simulink model "c00006M_harness"  (R2018a)
settings: Solver=FixedStepAuto  StartTime=0.0  StopTime=300  FixedStep=0.1  RelTol=1e-3
undefined symbols (not defined in the file): A1, hmax, PriorityTank, R1, R2, sigbuilder_block, TempThreshold
(part 19 of 66)

== system c00006M_harness/M091/Tank3/Control ==
  note: 1: Maintenance
      | 2: Reference
      | 3: Manual
  ControlType : Inport
  StartMaintenance : Inport  Port=2
  ManualReference : Inport  Port=3
  Fill : Inport  Port=4
  Empty : Inport  Port=5
  EmergencyButton : Inport  Port=6
  Temperature : Inport  Port=7
  LiquidLevel : Inport  Port=8
  Constant : Constant  Value=0
  Constant1 : Constant  Value=TempThreshold
  Logical Operator : Logic  Operator=OR  AllPortsSameDT=off  OutDataTypeStr=boolean
  Logical Operator1 : Logic  Operator=OR  AllPortsSameDT=off  OutDataTypeStr=boolean
  Maintenance : Subsystem
  ManualControlLiquidInOut : Subsystem
  ManualControlReference : Subsystem
  Multiport Switch : MultiPortSwitch
  Multiport Switch1 : MultiPortSwitch
  Relational Operator : RelationalOperator  Operator=>  OutDataTypeStr=boolean  RndMeth=Simplest
  Switch : Switch  Criteria=u2 > Threshold
  Switch1 : Switch  Criteria=u2 > Threshold
  LiquidIn : Outport
  LiquidOut : Outport  Port=2
  wires:
  Multiport Switch/1 -> Switch/3
  Multiport Switch1/1 -> Switch1/3
  ControlType/1 -> Multiport Switch1/1, Multiport Switch/1, Maintenance/1(Type)
  Maintenance/1(LiquidIn) -> Multiport Switch/2
  ManualControlReference/1(LiquidIn) -> Multiport Switch/3
  Maintenance/2(LiquidOut) -> Multiport Switch1/2
  ManualControlReference/2(LiquidOut) -> Multiport Switch1/3
  ManualReference/1 -> ManualControlReference/1(ManualReference)
  LiquidLevel/1 -> ManualControlLiquidInOut/3(LiquidLevel), ManualControlReference/2(LiquidLevel), Maintenance/3(LiquidLevel)
  ManualControlLiquidInOut/1(LiquidIn) -> Multiport Switch/4
  ManualControlLiquidInOut/2(LiquidOut) -> Multiport Switch1/4
  Empty/1 -> ManualControlLiquidInOut/2(Empty)
  Fill/1 -> ManualControlLiquidInOut/1(Fill)
  StartMaintenance/1 -> Maintenance/2(StartMaintenance)
  Switch/1 -> LiquidIn/1
  Switch1/1 -> LiquidOut/1
  Constant/1 -> Switch1/1, Switch/1
  EmergencyButton/1 -> Logical Operator/1, Logical Operator1/1
  Relational Operator/1 -> Logical Operator1/2, Logical Operator/2
  Logical Operator/1 -> Switch1/2
  Logical Operator1/1 -> Switch/2
  Temperature/1 -> Relational Operator/1
  Constant1/1 -> Relational Operator/2

== system c00006M_harness/M091/Tank3/MasterTankControl ==
  note: Priority tank must always have more liquid than others
  LiquidTank2 : Inport
  LiquidTank3 : Inport  Port=2
  Constant : Constant  Value=PriorityTank
  Constant1 : Constant  Value=false
  Logical Operator : Logic  Operator=NOT  AllPortsSameDT=off  OutDataTypeStr=boolean
  Multiport Switch : MultiPortSwitch
  Relational Operator1 : RelationalOperator  OutDataTypeStr=boolean  RndMeth=Simplest
  AllowTheTankFilling : Outport
  wires:
  Constant/1 -> Multiport Switch/1
  Relational Operator1/1 -> Multiport Switch/3
  Constant1/1 -> Multiport Switch/4, Multiport Switch/2
  Multiport Switch/1 -> Logical Operator/1
  Logical Operator/1 -> AllowTheTankFilling/1
  LiquidTank2/1 -> Relational Operator1/2
  LiquidTank3/1 -> Relational Operator1/1

== system c00006M_harness/M091/Tank3/TankModel ==
  LiquidIn : Inport
  LiquidOut : Inport  Port=2
  Add1 : Sum  Inputs=+-
  Constant1 : Constant  Value=0
  Constant2 : Constant  Value=0
  Constant3 : Constant
  Gain : Gain  Gain=1/R1
  Gain1 : Gain  Gain=1/A1
  Gain2 : Gain  Gain=1/R2
  Integrator : Integrator
  Saturation : Saturate  UpperLimit=hmax  LowerLimit=0
  Switch : Switch  Criteria=u2 ~= 0
  Switch1 : Switch  Criteria=u2 ~= 0
  LiquidLevel : Outport
  wires:
  Saturation/1 -> LiquidLevel/1, Gain2/1
  LiquidOut/1 -> Switch/2
  Add1/1 -> Gain1/1
  Gain2/1 -> Switch/1
  LiquidIn/1 -> Switch1/2
  Switch/1 -> Add1/2
  Switch1/1 -> Gain/1
  Constant2/1 -> Switch/3
  Constant3/1 -> Switch1/1
  Integrator/1 -> Saturation/1
  Gain1/1 -> Integrator/1
  Gain/1 -> Add1/1
  Constant1/1 -> Switch1/3

== system c00006M_harness/M092/Tank2/Control ==
  note: 1: Maintenance
      | 2: Reference
      | 3: Manual
  ControlType : Inport
  StartMaintenance : Inport  Port=2
  ManualReference : Inport  Port=3
  Fill : Inport  Port=4
  Empty : Inport  Port=5
  EmergencyButton : Inport  Port=6
  Temperature : Inport  Port=7
  LiquidLevel : Inport  Port=8
  Constant : Constant  Value=0
  Constant1 : Constant  Value=TempThreshold
  Logical Operator : Logic  Operator=OR  AllPortsSameDT=off  OutDataTypeStr=boolean
  Logical Operator1 : Logic  Operator=OR  AllPortsSameDT=off  OutDataTypeStr=boolean
  Maintenance : Subsystem
  ManualControlLiquidInOut : Subsystem
  ManualControlReference : Subsystem
  Multiport Switch : MultiPortSwitch
  Multiport Switch1 : MultiPortSwitch
  Relational Operator : RelationalOperator  Operator=>  OutDataTypeStr=boolean  RndMeth=Simplest
  Switch : Switch  Criteria=u2 > Threshold
  Switch1 : Switch  Criteria=u2 > Threshold
  LiquidIn : Outport
  LiquidOut : Outport  Port=2
  wires:
  Multiport Switch/1 -> Switch/3
  Multiport Switch1/1 -> Switch1/3
  ControlType/1 -> Multiport Switch1/1, Multiport Switch/1, Maintenance/1(Type)
  Maintenance/1(LiquidIn) -> Multiport Switch/2
  ManualControlReference/1(LiquidIn) -> Multiport Switch/3
  Maintenance/2(LiquidOut) -> Multiport Switch1/2
  ManualControlReference/2(LiquidOut) -> Multiport Switch1/3
  ManualReference/1 -> ManualControlReference/1(ManualReference)
  LiquidLevel/1 -> ManualControlLiquidInOut/3(LiquidLevel), ManualControlReference/2(LiquidLevel), Maintenance/3(LiquidLevel)
  ManualControlLiquidInOut/1(LiquidIn) -> Multiport Switch/4
  ManualControlLiquidInOut/2(LiquidOut) -> Multiport Switch1/4
  Empty/1 -> ManualControlLiquidInOut/2(Empty)
  Fill/1 -> ManualControlLiquidInOut/1(Fill)
  StartMaintenance/1 -> Maintenance/2(StartMaintenance)
  Switch/1 -> LiquidIn/1
  Switch1/1 -> LiquidOut/1
  Constant/1 -> Switch1/1, Switch/1
  EmergencyButton/1 -> Logical Operator/1, Logical Operator1/1
  Relational Operator/1 -> Logical Operator1/2, Logical Operator/2
  Logical Operator/1 -> Switch1/2
  Logical Operator1/1 -> Switch/2
  Temperature/1 -> Relational Operator/1
  Constant1/1 -> Relational Operator/2

== system c00006M_harness/M092/Tank2/MasterTankControl ==
  note: Priority tank must always have more liquid than others
  LiquidTank2 : Inport
  LiquidTank3 : Inport  Port=2
  Constant : Constant  Value=PriorityTank
  Constant1 : Constant  Value=false
  Logical Operator : Logic  Operator=NOT  AllPortsSameDT=off  OutDataTypeStr=boolean
  Multiport Switch : MultiPortSwitch
  Relational Operator1 : RelationalOperator  OutDataTypeStr=boolean  RndMeth=Simplest
  AllowTheTankFilling : Outport
  wires:
  LiquidTank2/1 -> Relational Operator1/1
  LiquidTank3/1 -> Relational Operator1/2
  Constant/1 -> Multiport Switch/1
  Relational Operator1/1 -> Multiport Switch/4
  Constant1/1 -> Multiport Switch/3, Multiport Switch/2
  Multiport Switch/1 -> Logical Operator/1
  Logical Operator/1 -> AllowTheTankFilling/1

== system c00006M_harness/M092/Tank2/TankModel ==
  LiquidIn : Inport
  LiquidOut : Inport  Port=2
  Add1 : Sum  Inputs=+-
  Constant1 : Constant  Value=0
  Constant2 : Constant  Value=0
  Constant3 : Constant
  Gain : Gain  Gain=1/R1
  Gain1 : Gain  Gain=1/A1
  Gain2 : Gain  Gain=1/R2
  Integrator : Integrator
  Saturation : Saturate  UpperLimit=hmax  LowerLimit=0
  Switch : Switch  Criteria=u2 ~= 0
  Switch1 : Switch  Criteria=u2 ~= 0
  LiquidLevel : Outport
  wires:
  Saturation/1 -> LiquidLevel/1, Gain2/1
  LiquidOut/1 -> Switch/2
  Add1/1 -> Gain1/1
  Gain2/1 -> Switch/1
  LiquidIn/1 -> Switch1/2
  Switch/1 -> Add1/2
  Switch1/1 -> Gain/1
  Constant2/1 -> Switch/3
  Constant3/1 -> Switch1/1
  Integrator/1 -> Saturation/1
  Gain1/1 -> Integrator/1
  Gain/1 -> Add1/1
  Constant1/1 -> Switch1/3

== system c00006M_harness/M092/Tank3/Control ==
  note: 1: Maintenance
      | 2: Reference
      | 3: Manual
  ControlType : Inport
  StartMaintenance : Inport  Port=2
  ManualReference : Inport  Port=3
  Fill : Inport  Port=4
  Empty : Inport  Port=5
  EmergencyButton : Inport  Port=6
  Temperature : Inport  Port=7
  LiquidLevel : Inport  Port=8
  Constant : Constant  Value=0
  Constant1 : Constant  Value=TempThreshold
  Logical Operator : Logic  Operator=OR  AllPortsSameDT=off  OutDataTypeStr=boolean
  Logical Operator1 : Logic  Operator=OR  AllPortsSameDT=off  OutDataTypeStr=boolean
  Maintenance : Subsystem
  ManualControlLiquidInOut : Subsystem
  ManualControlReference : Subsystem
  Multiport Switch : MultiPortSwitch
  Multiport Switch1 : MultiPortSwitch
  Relational Operator : RelationalOperator  Operator=>  OutDataTypeStr=boolean  RndMeth=Simplest
  Switch : Switch  Criteria=u2 > Threshold
  Switch1 : Switch  Criteria=u2 > Threshold
  LiquidIn : Outport
  LiquidOut : Outport  Port=2
  wires:
  Multiport Switch/1 -> Switch/3
  Multiport Switch1/1 -> Switch1/3
  ControlType/1 -> Multiport Switch1/1, Multiport Switch/1, Maintenance/1(Type)
  Maintenance/1(LiquidIn) -> Multiport Switch/2
  ManualControlReference/1(LiquidIn) -> Multiport Switch/3
  Maintenance/2(LiquidOut) -> Multiport Switch1/2
  ManualControlReference/2(LiquidOut) -> Multiport Switch1/3
  ManualReference/1 -> ManualControlReference/1(ManualReference)
  LiquidLevel/1 -> ManualControlLiquidInOut/3(LiquidLevel), ManualControlReference/2(LiquidLevel), Maintenance/3(LiquidLevel)
  ManualControlLiquidInOut/1(LiquidIn) -> Multiport Switch/4
  ManualControlLiquidInOut/2(LiquidOut) -> Multiport Switch1/4
  Empty/1 -> ManualControlLiquidInOut/2(Empty)
  Fill/1 -> ManualControlLiquidInOut/1(Fill)
  StartMaintenance/1 -> Maintenance/2(StartMaintenance)
  Switch/1 -> LiquidIn/1
  Switch1/1 -> LiquidOut/1
  Constant/1 -> Switch1/1, Switch/1
  EmergencyButton/1 -> Logical Operator/1, Logical Operator1/1
  Relational Operator/1 -> Logical Operator1/2, Logical Operator/2
  Logical Operator/1 -> Switch1/2
  Logical Operator1/1 -> Switch/2
  Temperature/1 -> Relational Operator/1
  Constant1/1 -> Relational Operator/2

== system c00006M_harness/M092/Tank3/MasterTankControl ==
  note: Priority tank must always have more liquid than others
  LiquidTank2 : Inport
  LiquidTank3 : Inport  Port=2
  Constant : Constant  Value=PriorityTank
  Constant1 : Constant  Value=false
  Logical Operator : Logic  Operator=NOT  AllPortsSameDT=off  OutDataTypeStr=boolean
  Multiport Switch : MultiPortSwitch
  Relational Operator1 : RelationalOperator  OutDataTypeStr=boolean  RndMeth=Simplest
  AllowTheTankFilling : Outport
  wires:
  Constant/1 -> Multiport Switch/1
  Relational Operator1/1 -> Multiport Switch/3
  Constant1/1 -> Multiport Switch/4, Multiport Switch/2
  Multiport Switch/1 -> Logical Operator/1
  Logical Operator/1 -> AllowTheTankFilling/1
  LiquidTank2/1 -> Relational Operator1/2
  LiquidTank3/1 -> Relational Operator1/1

== system c00006M_harness/M092/Tank3/TankModel ==
  LiquidIn : Inport
  LiquidOut : Inport  Port=2
  Add1 : Sum  Inputs=+-
  Constant1 : Constant  Value=0
  Constant2 : Constant  Value=0
  Constant3 : Constant
  Gain : Gain  Gain=1/R1
  Gain1 : Gain  Gain=1/A1
  Gain2 : Gain  Gain=1/R2
  Integrator : Integrator
  Saturation : Saturate  UpperLimit=hmax  LowerLimit=0
  Switch : Switch  Criteria=u2 ~= 0
  Switch1 : Switch  Criteria=u2 ~= 0
  LiquidLevel : Outport
  wires:
  Saturation/1 -> LiquidLevel/1, Gain2/1
  LiquidOut/1 -> Switch/2
  Add1/1 -> Gain1/1
  Gain2/1 -> Switch/1
  LiquidIn/1 -> Switch1/2
  Switch/1 -> Add1/2
  Switch1/1 -> Gain/1
  Constant2/1 -> Switch/3
  Constant3/1 -> Switch1/1
  Integrator/1 -> Saturation/1
  Gain1/1 -> Integrator/1
  Gain/1 -> Add1/1
  Constant1/1 -> Switch1/3

== system c00006M_harness/M093/Tank2/Control ==
  note: 1: Maintenance
      | 2: Reference
      | 3: Manual
  ControlType : Inport
  StartMaintenance : Inport  Port=2
  ManualReference : Inport  Port=3
  Fill : Inport  Port=4
  Empty : Inport  Port=5
  EmergencyButton : Inport  Port=6
  Temperature : Inport  Port=7
  LiquidLevel : Inport  Port=8
  Constant : Constant  Value=0
  Constant1 : Constant  Value=TempThreshold
  Logical Operator : Logic  Operator=OR  AllPortsSameDT=off  OutDataTypeStr=boolean
  Logical Operator1 : Logic  Operator=OR  AllPortsSameDT=off  OutDataTypeStr=boolean
  Maintenance : Subsystem
  ManualControlLiquidInOut : Subsystem
  ManualControlReference : Subsystem
  Multiport Switch : MultiPortSwitch
  Multiport Switch1 : MultiPortSwitch
  Relational Operator : RelationalOperator  Operator=>  OutDataTypeStr=boolean  RndMeth=Simplest
  Switch : Switch  Criteria=u2 > Threshold
  Switch1 : Switch  Criteria=u2 > Threshold
  LiquidIn : Outport
  LiquidOut : Outport  Port=2
  wires:
  Multiport Switch/1 -> Switch/3
  Multiport Switch1/1 -> Switch1/3
  ControlType/1 -> Multiport Switch1/1, Multiport Switch/1, Maintenance/1(Type)
  Maintenance/1(LiquidIn) -> Multiport Switch/2
  ManualControlReference/1(LiquidIn) -> Multiport Switch/3
  Maintenance/2(LiquidOut) -> Multiport Switch1/2
  ManualControlReference/2(LiquidOut) -> Multiport Switch1/3
  ManualReference/1 -> ManualControlReference/1(ManualReference)
  LiquidLevel/1 -> ManualControlLiquidInOut/3(LiquidLevel), ManualControlReference/2(LiquidLevel), Maintenance/3(LiquidLevel)
  ManualControlLiquidInOut/1(LiquidIn) -> Multiport Switch/4
  ManualControlLiquidInOut/2(LiquidOut) -> Multiport Switch1/4
  Empty/1 -> ManualControlLiquidInOut/2(Empty)
  Fill/1 -> ManualControlLiquidInOut/1(Fill)
  StartMaintenance/1 -> Maintenance/2(StartMaintenance)
  Switch/1 -> LiquidIn/1
  Switch1/1 -> LiquidOut/1
  Constant/1 -> Switch1/1, Switch/1
  EmergencyButton/1 -> Logical Operator/1, Logical Operator1/1
  Relational Operator/1 -> Logical Operator1/2, Logical Operator/2
  Logical Operator/1 -> Switch1/2
  Logical Operator1/1 -> Switch/2
  Temperature/1 -> Relational Operator/1
  Constant1/1 -> Relational Operator/2

== system c00006M_harness/M093/Tank2/MasterTankControl ==
  note: Priority tank must always have more liquid than others
  LiquidTank2 : Inport
  LiquidTank3 : Inport  Port=2
  Constant : Constant  Value=PriorityTank
  Constant1 : Constant  Value=false
  Logical Operator : Logic  Operator=NOT  AllPortsSameDT=off  OutDataTypeStr=boolean
  Multiport Switch : MultiPortSwitch
  Relational Operator1 : RelationalOperator  OutDataTypeStr=boolean  RndMeth=Simplest
  AllowTheTankFilling : Outport
  wires:
  LiquidTank2/1 -> Relational Operator1/1
  LiquidTank3/1 -> Relational Operator1/2
  Constant/1 -> Multiport Switch/1
  Relational Operator1/1 -> Multiport Switch/4
  Constant1/1 -> Multiport Switch/3, Multiport Switch/2
  Multiport Switch/1 -> Logical Operator/1
  Logical Operator/1 -> AllowTheTankFilling/1

== system c00006M_harness/M093/Tank2/TankModel ==
  LiquidIn : Inport
  LiquidOut : Inport  Port=2
  Add1 : Sum  Inputs=+-
  Constant1 : Constant  Value=0
  Constant2 : Constant  Value=0
  Constant3 : Constant
  Gain : Gain  Gain=1/R1
  Gain1 : Gain  Gain=1/A1
  Gain2 : Gain  Gain=1/R2
  Integrator : Integrator
  Saturation : Saturate  UpperLimit=hmax  LowerLimit=0
  Switch : Switch  Criteria=u2 ~= 0
  Switch1 : Switch  Criteria=u2 ~= 0
  LiquidLevel : Outport
  wires:
  Saturation/1 -> LiquidLevel/1, Gain2/1
  LiquidOut/1 -> Switch/2
  Add1/1 -> Gain1/1
  Gain2/1 -> Switch/1
  LiquidIn/1 -> Switch1/2
  Switch/1 -> Add1/2
  Switch1/1 -> Gain/1
  Constant2/1 -> Switch/3
  Constant3/1 -> Switch1/1
  Integrator/1 -> Saturation/1
  Gain1/1 -> Integrator/1
  Gain/1 -> Add1/1
  Constant1/1 -> Switch1/3

== system c00006M_harness/M093/Tank3/Control ==
  note: 1: Maintenance
      | 2: Reference
      | 3: Manual
  ControlType : Inport
  StartMaintenance : Inport  Port=2
  ManualReference : Inport  Port=3
  Fill : Inport  Port=4
  Empty : Inport  Port=5
  EmergencyButton : Inport  Port=6
  Temperature : Inport  Port=7
  LiquidLevel : Inport  Port=8
  Constant : Constant  Value=0
  Constant1 : Constant  Value=TempThreshold
  Logical Operator : Logic  Operator=OR  AllPortsSameDT=off  OutDataTypeStr=boolean
  Logical Operator1 : Logic  Operator=OR  AllPortsSameDT=off  OutDataTypeStr=boolean
  Maintenance : Subsystem
  ManualControlLiquidInOut : Subsystem
  ManualControlReference : Subsystem
  Multiport Switch : MultiPortSwitch
  Multiport Switch1 : MultiPortSwitch
  Relational Operator : RelationalOperator  Operator=>  OutDataTypeStr=boolean  RndMeth=Simplest
  Switch : Switch  Criteria=u2 > Threshold
  Switch1 : Switch  Criteria=u2 > Threshold
  LiquidIn : Outport
  LiquidOut : Outport  Port=2
  wires:
  Multiport Switch/1 -> Switch/3
  Multiport Switch1/1 -> Switch1/3
  ControlType/1 -> Multiport Switch1/1, Multiport Switch/1, Maintenance/1(Type)
  Maintenance/1(LiquidIn) -> Multiport Switch/2
  ManualControlReference/1(LiquidIn) -> Multiport Switch/3
  Maintenance/2(LiquidOut) -> Multiport Switch1/2
  ManualControlReference/2(LiquidOut) -> Multiport Switch1/3
  ManualReference/1 -> ManualControlReference/1(ManualReference)
  LiquidLevel/1 -> ManualControlLiquidInOut/3(LiquidLevel), ManualControlReference/2(LiquidLevel), Maintenance/3(LiquidLevel)
  ManualControlLiquidInOut/1(LiquidIn) -> Multiport Switch/4
  ManualControlLiquidInOut/2(LiquidOut) -> Multiport Switch1/4
  Empty/1 -> ManualControlLiquidInOut/2(Empty)
  Fill/1 -> ManualControlLiquidInOut/1(Fill)
  StartMaintenance/1 -> Maintenance/2(StartMaintenance)
  Switch/1 -> LiquidIn/1
  Switch1/1 -> LiquidOut/1
  Constant/1 -> Switch1/1, Switch/1
  EmergencyButton/1 -> Logical Operator/1, Logical Operator1/1
  Relational Operator/1 -> Logical Operator1/2, Logical Operator/2
  Logical Operator/1 -> Switch1/2
  Logical Operator1/1 -> Switch/2
  Temperature/1 -> Relational Operator/1
  Constant1/1 -> Relational Operator/2

== system c00006M_harness/M093/Tank3/MasterTankControl ==
  note: Priority tank must always have more liquid than others
  LiquidTank2 : Inport
  LiquidTank3 : Inport  Port=2
  Constant : Constant  Value=PriorityTank
  Constant1 : Constant  Value=false
  Logical Operator : Logic  Operator=NOT  AllPortsSameDT=off  OutDataTypeStr=boolean
  Multiport Switch : MultiPortSwitch
  Relational Operator1 : RelationalOperator  OutDataTypeStr=boolean  RndMeth=Simplest
  AllowTheTankFilling : Outport
  wires:
  Constant/1 -> Multiport Switch/1
  Relational Operator1/1 -> Multiport Switch/3
  Constant1/1 -> Multiport Switch/4, Multiport Switch/2
  Multiport Switch/1 -> Logical Operator/1
  Logical Operator/1 -> AllowTheTankFilling/1
  LiquidTank2/1 -> Relational Operator1/2
  LiquidTank3/1 -> Relational Operator1/1

== system c00006M_harness/M093/Tank3/TankModel ==
  LiquidIn : Inport
  LiquidOut : Inport  Port=2
  Add1 : Sum  Inputs=+-
  Constant1 : Constant  Value=0
  Constant2 : Constant  Value=0
  Constant3 : Constant
  Gain : Gain  Gain=1/R1
  Gain1 : Gain  Gain=1/A1
  Gain2 : Gain  Gain=1/R2
  Integrator : Integrator
  Saturation : Saturate  UpperLimit=hmax  LowerLimit=0
  Switch : Switch  Criteria=u2 ~= 0
  Switch1 : Switch  Criteria=u2 ~= 0
  LiquidLevel : Outport
  wires:
  Saturation/1 -> LiquidLevel/1, Gain2/1
  LiquidOut/1 -> Switch/2
  Add1/1 -> Gain1/1
  Gain2/1 -> Switch/1
  LiquidIn/1 -> Switch1/2
  Switch/1 -> Add1/2
  Switch1/1 -> Gain/1
  Constant2/1 -> Switch/3
  Constant3/1 -> Switch1/1
  Integrator/1 -> Saturation/1
  Gain1/1 -> Integrator/1
  Gain/1 -> Add1/1
  Constant1/1 -> Switch1/3

== system c00006M_harness/M094/Tank2/Control ==
  note: 1: Maintenance
      | 2: Reference
      | 3: Manual
  ControlType : Inport
  StartMaintenance : Inport  Port=2
  ManualReference : Inport  Port=3
  Fill : Inport  Port=4
  Empty : Inport  Port=5
  EmergencyButton : Inport  Port=6
  Temperature : Inport  Port=7
  LiquidLevel : Inport  Port=8
  Constant : Constant  Value=0
  Constant1 : Constant  Value=TempThreshold
  Logical Operator : Logic  Operator=OR  AllPortsSameDT=off  OutDataTypeStr=boolean
  Logical Operator1 : Logic  Operator=OR  AllPortsSameDT=off  OutDataTypeStr=boolean
  Maintenance : Subsystem
  ManualControlLiquidInOut : Subsystem
  ManualControlReference : Subsystem
  Multiport Switch : MultiPortSwitch
  Multiport Switch1 : MultiPortSwitch
  Relational Operator : RelationalOperator  Operator=>  OutDataTypeStr=boolean  RndMeth=Simplest
  Switch : Switch  Criteria=u2 > Threshold
  Switch1 : Switch  Criteria=u2 > Threshold
  LiquidIn : Outport
  LiquidOut : Outport  Port=2
  wires:
  Multiport Switch/1 -> Switch/3
  Multiport Switch1/1 -> Switch1/3
  ControlType/1 -> Multiport Switch1/1, Multiport Switch/1, Maintenance/1(Type)
  Maintenance/1(LiquidIn) -> Multiport Switch/2
  ManualControlReference/1(LiquidIn) -> Multiport Switch/3
  Maintenance/2(LiquidOut) -> Multiport Switch1/2
  ManualControlReference/2(LiquidOut) -> Multiport Switch1/3
  ManualReference/1 -> ManualControlReference/1(ManualReference)
  LiquidLevel/1 -> ManualControlLiquidInOut/3(LiquidLevel), ManualControlReference/2(LiquidLevel), Maintenance/3(LiquidLevel)
  ManualControlLiquidInOut/1(LiquidIn) -> Multiport Switch/4
  ManualControlLiquidInOut/2(LiquidOut) -> Multiport Switch1/4
  Empty/1 -> ManualControlLiquidInOut/2(Empty)
  Fill/1 -> ManualControlLiquidInOut/1(Fill)
  StartMaintenance/1 -> Maintenance/2(StartMaintenance)
  Switch/1 -> LiquidIn/1
  Switch1/1 -> LiquidOut/1
  Constant/1 -> Switch1/1, Switch/1
  EmergencyButton/1 -> Logical Operator/1, Logical Operator1/1
  Relational Operator/1 -> Logical Operator1/2, Logical Operator/2
  Logical Operator/1 -> Switch1/2
  Logical Operator1/1 -> Switch/2
  Temperature/1 -> Relational Operator/1
  Constant1/1 -> Relational Operator/2

== system c00006M_harness/M094/Tank2/MasterTankControl ==
  note: Priority tank must always have more liquid than others
  LiquidTank2 : Inport
  LiquidTank3 : Inport  Port=2
  Constant : Constant  Value=PriorityTank
  Constant1 : Constant  Value=false
  Logical Operator : Logic  Operator=NOT  AllPortsSameDT=off  OutDataTypeStr=boolean
  Multiport Switch : MultiPortSwitch
  Relational Operator1 : RelationalOperator  OutDataTypeStr=boolean  RndMeth=Simplest
  AllowTheTankFilling : Outport
  wires:
  LiquidTank2/1 -> Relational Operator1/1
  LiquidTank3/1 -> Relational Operator1/2
  Constant/1 -> Multiport Switch/1
  Relational Operator1/1 -> Multiport Switch/4
  Constant1/1 -> Multiport Switch/3, Multiport Switch/2
  Multiport Switch/1 -> Logical Operator/1
  Logical Operator/1 -> AllowTheTankFilling/1

== system c00006M_harness/M094/Tank2/TankModel ==
  LiquidIn : Inport
  LiquidOut : Inport  Port=2
  Add1 : Sum  Inputs=+-
  Constant1 : Constant  Value=0
  Constant2 : Constant  Value=0
  Constant3 : Constant
  Gain : Gain  Gain=1/R1
  Gain1 : Gain  Gain=1/A1
  Gain2 : Gain  Gain=1/R2
  Integrator : Integrator
  Saturation : Saturate  UpperLimit=hmax  LowerLimit=0
  Switch : Switch  Criteria=u2 ~= 0
  Switch1 : Switch  Criteria=u2 ~= 0
  LiquidLevel : Outport
  wires:
  Saturation/1 -> LiquidLevel/1, Gain2/1
  LiquidOut/1 -> Switch/2
  Add1/1 -> Gain1/1
  Gain2/1 -> Switch/1
  LiquidIn/1 -> Switch1/2
  Switch/1 -> Add1/2
  Switch1/1 -> Gain/1
  Constant2/1 -> Switch/3
  Constant3/1 -> Switch1/1
  Integrator/1 -> Saturation/1
  Gain1/1 -> Integrator/1
  Gain/1 -> Add1/1
  Constant1/1 -> Switch1/3

== system c00006M_harness/M094/Tank3/Control ==
  note: 1: Maintenance
      | 2: Reference
      | 3: Manual
  ControlType : Inport
  StartMaintenance : Inport  Port=2
  ManualReference : Inport  Port=3
  Fill : Inport  Port=4
  Empty : Inport  Port=5
  EmergencyButton : Inport  Port=6
  Temperature : Inport  Port=7
  LiquidLevel : Inport  Port=8
  Constant : Constant  Value=0
  Constant1 : Constant  Value=TempThreshold
  Logical Operator : Logic  Operator=OR  AllPortsSameDT=off  OutDataTypeStr=boolean
  Logical Operator1 : Logic  Operator=OR  AllPortsSameDT=off  OutDataTypeStr=boolean
  Maintenance : Subsystem
  ManualControlLiquidInOut : Subsystem
  ManualControlReference : Subsystem
  Multiport Switch : MultiPortSwitch
  Multiport Switch1 : MultiPortSwitch
  Relational Operator : RelationalOperator  Operator=>  OutDataTypeStr=boolean  RndMeth=Simplest
  Switch : Switch  Criteria=u2 > Threshold
  Switch1 : Switch  Criteria=u2 > Threshold
  LiquidIn : Outport
  LiquidOut : Outport  Port=2
  wires:
  Multiport Switch/1 -> Switch/3
  Multiport Switch1/1 -> Switch1/3
  ControlType/1 -> Multiport Switch1/1, Multiport Switch/1, Maintenance/1(Type)
  Maintenance/1(LiquidIn) -> Multiport Switch/2
  ManualControlReference/1(LiquidIn) -> Multiport Switch/3
  Maintenance/2(LiquidOut) -> Multiport Switch1/2
  ManualControlReference/2(LiquidOut) -> Multiport Switch1/3
  ManualReference/1 -> ManualControlReference/1(ManualReference)
  LiquidLevel/1 -> ManualControlLiquidInOut/3(LiquidLevel), ManualControlReference/2(LiquidLevel), Maintenance/3(LiquidLevel)
  ManualControlLiquidInOut/1(LiquidIn) -> Multiport Switch/4
  ManualControlLiquidInOut/2(LiquidOut) -> Multiport Switch1/4
  Empty/1 -> ManualControlLiquidInOut/2(Empty)
  Fill/1 -> ManualControlLiquidInOut/1(Fill)
  StartMaintenance/1 -> Maintenance/2(StartMaintenance)
  Switch/1 -> LiquidIn/1
  Switch1/1 -> LiquidOut/1
  Constant/1 -> Switch1/1, Switch/1
  EmergencyButton/1 -> Logical Operator/1, Logical Operator1/1
  Relational Operator/1 -> Logical Operator1/2, Logical Operator/2
  Logical Operator/1 -> Switch1/2
  Logical Operator1/1 -> Switch/2
  Temperature/1 -> Relational Operator/1
  Constant1/1 -> Relational Operator/2

== system c00006M_harness/M094/Tank3/MasterTankControl ==
  note: Priority tank must always have more liquid than others
  LiquidTank2 : Inport
  LiquidTank3 : Inport  Port=2
  Constant : Constant  Value=PriorityTank
  Constant1 : Constant  Value=false
  Logical Operator : Logic  Operator=NOT  AllPortsSameDT=off  OutDataTypeStr=boolean
  Multiport Switch : MultiPortSwitch
  Relational Operator1 : RelationalOperator  OutDataTypeStr=boolean  RndMeth=Simplest
  AllowTheTankFilling : Outport
  wires:
  Constant/1 -> Multiport Switch/1
  Relational Operator1/1 -> Multiport Switch/3
  Constant1/1 -> Multiport Switch/4, Multiport Switch/2
  Multiport Switch/1 -> Logical Operator/1
  Logical Operator/1 -> AllowTheTankFilling/1
  LiquidTank2/1 -> Relational Operator1/2
  LiquidTank3/1 -> Relational Operator1/1

== system c00006M_harness/M094/Tank3/TankModel ==
  LiquidIn : Inport
  LiquidOut : Inport  Port=2
  Add1 : Sum  Inputs=+-
  Constant1 : Constant  Value=0
  Constant2 : Constant  Value=0
  Constant3 : Constant
  Gain : Gain  Gain=1/R1
  Gain1 : Gain  Gain=1/A1
  Gain2 : Gain  Gain=1/R2
  Integrator : Integrator
  Saturation : Saturate  UpperLimit=hmax  LowerLimit=0
  Switch : Switch  Criteria=u2 ~= 0
  Switch1 : Switch  Criteria=u2 ~= 0
  LiquidLevel : Outport
  wires:
  Saturation/1 -> LiquidLevel/1, Gain2/1
  LiquidOut/1 -> Switch/2
  Add1/1 -> Gain1/1
  Gain2/1 -> Switch/1
  LiquidIn/1 -> Switch1/2
  Switch/1 -> Add1/2
  Switch1/1 -> Gain/1
  Constant2/1 -> Switch/3
  Constant3/1 -> Switch1/1
  Integrator/1 -> Saturation/1
  Gain1/1 -> Integrator/1
  Gain/1 -> Add1/1
  Constant1/1 -> Switch1/3

== system c00006M_harness/M095/Tank2/Control ==
  note: 1: Maintenance
      | 2: Reference
      | 3: Manual
  ControlType : Inport
  StartMaintenance : Inport  Port=2
  ManualReference : Inport  Port=3
  Fill : Inport  Port=4
  Empty : Inport  Port=5
  EmergencyButton : Inport  Port=6
  Temperature : Inport  Port=7
  LiquidLevel : Inport  Port=8
  Constant : Constant  Value=0
  Constant1 : Constant  Value=TempThreshold
  Logical Operator : Logic  Operator=OR  AllPortsSameDT=off  OutDataTypeStr=boolean
  Logical Operator1 : Logic  Operator=OR  AllPortsSameDT=off  OutDataTypeStr=boolean
  Maintenance : Subsystem
  ManualControlLiquidInOut : Subsystem
  ManualControlReference : Subsystem
  Multiport Switch : MultiPortSwitch
  Multiport Switch1 : MultiPortSwitch
  Relational Operator : RelationalOperator  Operator=>  OutDataTypeStr=boolean  RndMeth=Simplest
  Switch : Switch  Criteria=u2 > Threshold
  Switch1 : Switch  Criteria=u2 > Threshold
  LiquidIn : Outport
  LiquidOut : Outport  Port=2
  wires:
  Multiport Switch/1 -> Switch/3
  Multiport Switch1/1 -> Switch1/3
  ControlType/1 -> Multiport Switch1/1, Multiport Switch/1, Maintenance/1(Type)
  Maintenance/1(LiquidIn) -> Multiport Switch/2
  ManualControlReference/1(LiquidIn) -> Multiport Switch/3
  Maintenance/2(LiquidOut) -> Multiport Switch1/2
  ManualControlReference/2(LiquidOut) -> Multiport Switch1/3
  ManualReference/1 -> ManualControlReference/1(ManualReference)
  LiquidLevel/1 -> ManualControlLiquidInOut/3(LiquidLevel), ManualControlReference/2(LiquidLevel), Maintenance/3(LiquidLevel)
  ManualControlLiquidInOut/1(LiquidIn) -> Multiport Switch/4
  ManualControlLiquidInOut/2(LiquidOut) -> Multiport Switch1/4
  Empty/1 -> ManualControlLiquidInOut/2(Empty)
  Fill/1 -> ManualControlLiquidInOut/1(Fill)
  StartMaintenance/1 -> Maintenance/2(StartMaintenance)
  Switch/1 -> LiquidIn/1
  Switch1/1 -> LiquidOut/1
  Constant/1 -> Switch1/1, Switch/1
  EmergencyButton/1 -> Logical Operator/1, Logical Operator1/1
  Relational Operator/1 -> Logical Operator1/2, Logical Operator/2
  Logical Operator/1 -> Switch1/2
  Logical Operator1/1 -> Switch/2
  Temperature/1 -> Relational Operator/1
  Constant1/1 -> Relational Operator/2

== system c00006M_harness/M095/Tank2/MasterTankControl ==
  note: Priority tank must always have more liquid than others
  LiquidTank2 : Inport
  LiquidTank3 : Inport  Port=2
  Constant : Constant  Value=PriorityTank
  Constant1 : Constant  Value=false
  Logical Operator : Logic  Operator=NOT  AllPortsSameDT=off  OutDataTypeStr=boolean
  Multiport Switch : MultiPortSwitch
  Relational Operator1 : RelationalOperator  OutDataTypeStr=boolean  RndMeth=Simplest
  AllowTheTankFilling : Outport
  wires:
  LiquidTank2/1 -> Relational Operator1/1
  LiquidTank3/1 -> Relational Operator1/2
  Constant/1 -> Multiport Switch/1
  Relational Operator1/1 -> Multiport Switch/4
  Constant1/1 -> Multiport Switch/3, Multiport Switch/2
  Multiport Switch/1 -> Logical Operator/1
  Logical Operator/1 -> AllowTheTankFilling/1

== system c00006M_harness/M095/Tank2/TankModel ==
  LiquidIn : Inport
  LiquidOut : Inport  Port=2
  Add1 : Sum  Inputs=+-
  Constant1 : Constant  Value=0
  Constant2 : Constant  Value=0
  Constant3 : Constant
  Gain : Gain  Gain=1/R1
  Gain1 : Gain  Gain=1/A1
  Gain2 : Gain  Gain=1/R2
  Integrator : Integrator
  Saturation : Saturate  UpperLimit=hmax  LowerLimit=0
  Switch : Switch  Criteria=u2 ~= 0
  Switch1 : Switch  Criteria=u2 ~= 0
  LiquidLevel : Outport
  wires:
  Saturation/1 -> LiquidLevel/1, Gain2/1
  LiquidOut/1 -> Switch/2
  Add1/1 -> Gain1/1
  Gain2/1 -> Switch/1
  LiquidIn/1 -> Switch1/2
  Switch/1 -> Add1/2
  Switch1/1 -> Gain/1
  Constant2/1 -> Switch/3
  Constant3/1 -> Switch1/1
  Integrator/1 -> Saturation/1
  Gain1/1 -> Integrator/1
  Gain/1 -> Add1/1
  Constant1/1 -> Switch1/3

== system c00006M_harness/M095/Tank3/Control ==
  note: 1: Maintenance
      | 2: Reference
      | 3: Manual
  ControlType : Inport
  StartMaintenance : Inport  Port=2
  ManualReference : Inport  Port=3
  Fill : Inport  Port=4
  Empty : Inport  Port=5
  EmergencyButton : Inport  Port=6
  Temperature : Inport  Port=7
  LiquidLevel : Inport  Port=8
  Constant : Constant  Value=0
  Constant1 : Constant  Value=TempThreshold
  Logical Operator : Logic  Operator=OR  AllPortsSameDT=off  OutDataTypeStr=boolean
  Logical Operator1 : Logic  Operator=OR  AllPortsSameDT=off  OutDataTypeStr=boolean
  Maintenance : Subsystem
  ManualControlLiquidInOut : Subsystem
  ManualControlReference : Subsystem
  Multiport Switch : MultiPortSwitch
  Multiport Switch1 : MultiPortSwitch
  Relational Operator : RelationalOperator  Operator=>  OutDataTypeStr=boolean  RndMeth=Simplest
  Switch : Switch  Criteria=u2 > Threshold
  Switch1 : Switch  Criteria=u2 > Threshold
  LiquidIn : Outport
  LiquidOut : Outport  Port=2
  wires:
  Multiport Switch/1 -> Switch/3
  Multiport Switch1/1 -> Switch1/3
  ControlType/1 -> Multiport Switch1/1, Multiport Switch/1, Maintenance/1(Type)
  Maintenance/1(LiquidIn) -> Multiport Switch/2
  ManualControlReference/1(LiquidIn) -> Multiport Switch/3
  Maintenance/2(LiquidOut) -> Multiport Switch1/2
  ManualControlReference/2(LiquidOut) -> Multiport Switch1/3
  ManualReference/1 -> ManualControlReference/1(ManualReference)
  LiquidLevel/1 -> ManualControlLiquidInOut/3(LiquidLevel), ManualControlReference/2(LiquidLevel), Maintenance/3(LiquidLevel)
  ManualControlLiquidInOut/1(LiquidIn) -> Multiport Switch/4
  ManualControlLiquidInOut/2(LiquidOut) -> Multiport Switch1/4
  Empty/1 -> ManualControlLiquidInOut/2(Empty)
  Fill/1 -> ManualControlLiquidInOut/1(Fill)
  StartMaintenance/1 -> Maintenance/2(StartMaintenance)
  Switch/1 -> LiquidIn/1
  Switch1/1 -> LiquidOut/1
  Constant/1 -> Switch1/1, Switch/1
  EmergencyButton/1 -> Logical Operator/1, Logical Operator1/1
  Relational Operator/1 -> Logical Operator1/2, Logical Operator/2
  Logical Operator/1 -> Switch1/2
  Logical Operator1/1 -> Switch/2
  Temperature/1 -> Relational Operator/1
  Constant1/1 -> Relational Operator/2

== system c00006M_harness/M095/Tank3/MasterTankControl ==
  note: Priority tank must always have more liquid than others
  LiquidTank2 : Inport
  LiquidTank3 : Inport  Port=2
  Constant : Constant  Value=PriorityTank
  Constant1 : Constant  Value=false
  Logical Operator : Logic  Operator=NOT  AllPortsSameDT=off  OutDataTypeStr=boolean
  Multiport Switch : MultiPortSwitch
  Relational Operator1 : RelationalOperator  OutDataTypeStr=boolean  RndMeth=Simplest
  AllowTheTankFilling : Outport
  wires:
  Constant/1 -> Multiport Switch/1
  Relational Operator1/1 -> Multiport Switch/3
  Constant1/1 -> Multiport Switch/4, Multiport Switch/2
  Multiport Switch/1 -> Logical Operator/1
  Logical Operator/1 -> AllowTheTankFilling/1
  LiquidTank2/1 -> Relational Operator1/2
  LiquidTank3/1 -> Relational Operator1/1

== system c00006M_harness/M095/Tank3/TankModel ==
  LiquidIn : Inport
  LiquidOut : Inport  Port=2
  Add1 : Sum  Inputs=+-
  Constant1 : Constant  Value=0
  Constant2 : Constant  Value=0
  Constant3 : Constant
  Gain : Gain  Gain=1/R1
  Gain1 : Gain  Gain=1/A1
  Gain2 : Gain  Gain=1/R2
  Integrator : Integrator
  Saturation : Saturate  UpperLimit=hmax  LowerLimit=0
  Switch : Switch  Criteria=u2 ~= 0
  Switch1 : Switch  Criteria=u2 ~= 0
  LiquidLevel : Outport
  wires:
  Saturation/1 -> LiquidLevel/1, Gain2/1
  LiquidOut/1 -> Switch/2
  Add1/1 -> Gain1/1
  Gain2/1 -> Switch/1
  LiquidIn/1 -> Switch1/2
  Switch/1 -> Add1/2
  Switch1/1 -> Gain/1
  Constant2/1 -> Switch/3
  Constant3/1 -> Switch1/1
  Integrator/1 -> Saturation/1
  Gain1/1 -> Integrator/1
  Gain/1 -> Add1/1
  Constant1/1 -> Switch1/3

== system c00006M_harness/M096/Tank2/Control ==
  note: 1: Maintenance
      | 2: Reference
      | 3: Manual
  ControlType : Inport
  StartMaintenance : Inport  Port=2
  ManualReference : Inport  Port=3
  Fill : Inport  Port=4
  Empty : Inport  Port=5
  EmergencyButton : Inport  Port=6
  Temperature : Inport  Port=7
  LiquidLevel : Inport  Port=8
  Constant : Constant  Value=0
  Constant1 : Constant  Value=TempThreshold
  Logical Operator : Logic  Operator=OR  AllPortsSameDT=off  OutDataTypeStr=boolean
  Logical Operator1 : Logic  Operator=OR  AllPortsSameDT=off  OutDataTypeStr=boolean
  Maintenance : Subsystem
  ManualControlLiquidInOut : Subsystem
  ManualControlReference : Subsystem
  Multiport Switch : MultiPortSwitch
  Multiport Switch1 : MultiPortSwitch
  Relational Operator : RelationalOperator  Operator=>  OutDataTypeStr=boolean  RndMeth=Simplest
  Switch : Switch  Criteria=u2 > Threshold
  Switch1 : Switch  Criteria=u2 > Threshold
  LiquidIn : Outport
  LiquidOut : Outport  Port=2
  wires:
  Multiport Switch/1 -> Switch/3
  Multiport Switch1/1 -> Switch1/3
  ControlType/1 -> Multiport Switch1/1, Multiport Switch/1, Maintenance/1(Type)
  Maintenance/1(LiquidIn) -> Multiport Switch/2
  ManualControlReference/1(LiquidIn) -> Multiport Switch/3
  Maintenance/2(LiquidOut) -> Multiport Switch1/2
  ManualControlReference/2(LiquidOut) -> Multiport Switch1/3
  ManualReference/1 -> ManualControlReference/1(ManualReference)
  LiquidLevel/1 -> ManualControlLiquidInOut/3(LiquidLevel), ManualControlReference/2(LiquidLevel), Maintenance/3(LiquidLevel)
  ManualControlLiquidInOut/1(LiquidIn) -> Multiport Switch/4
  ManualControlLiquidInOut/2(LiquidOut) -> Multiport Switch1/4
  Empty/1 -> ManualControlLiquidInOut/2(Empty)
  Fill/1 -> ManualControlLiquidInOut/1(Fill)
  StartMaintenance/1 -> Maintenance/2(StartMaintenance)
  Switch/1 -> LiquidIn/1
  Switch1/1 -> LiquidOut/1
  Constant/1 -> Switch1/1, Switch/1
  EmergencyButton/1 -> Logical Operator/1, Logical Operator1/1
  Relational Operator/1 -> Logical Operator1/2, Logical Operator/2
  Logical Operator/1 -> Switch1/2
  Logical Operator1/1 -> Switch/2
  Temperature/1 -> Relational Operator/1
  Constant1/1 -> Relational Operator/2

== system c00006M_harness/M096/Tank2/MasterTankControl ==
  note: Priority tank must always have more liquid than others
  LiquidTank2 : Inport
  LiquidTank3 : Inport  Port=2
  Constant : Constant  Value=PriorityTank
  Constant1 : Constant  Value=false
  Logical Operator : Logic  Operator=NOT  AllPortsSameDT=off  OutDataTypeStr=boolean
  Multiport Switch : MultiPortSwitch
  Relational Operator1 : RelationalOperator  OutDataTypeStr=boolean  RndMeth=Simplest
  AllowTheTankFilling : Outport
  wires:
  LiquidTank2/1 -> Relational Operator1/1
  LiquidTank3/1 -> Relational Operator1/2
  Constant/1 -> Multiport Switch/1
  Relational Operator1/1 -> Multiport Switch/4
  Constant1/1 -> Multiport Switch/3, Multiport Switch/2
  Multiport Switch/1 -> Logical Operator/1
  Logical Operator/1 -> AllowTheTankFilling/1

== system c00006M_harness/M096/Tank2/TankModel ==
  LiquidIn : Inport
  LiquidOut : Inport  Port=2
  Add1 : Sum  Inputs=+-
  Constant1 : Constant  Value=0
  Constant2 : Constant  Value=0
  Constant3 : Constant
  Gain : Gain  Gain=1/R1
  Gain1 : Gain  Gain=1/A1
  Gain2 : Gain  Gain=1/R2
  Integrator : Integrator
  Saturation : Saturate  UpperLimit=hmax  LowerLimit=0
  Switch : Switch  Criteria=u2 ~= 0
  Switch1 : Switch  Criteria=u2 ~= 0
  LiquidLevel : Outport
  wires:
  Saturation/1 -> LiquidLevel/1, Gain2/1
  LiquidOut/1 -> Switch/2
  Add1/1 -> Gain1/1
  Gain2/1 -> Switch/1
  LiquidIn/1 -> Switch1/2
  Switch/1 -> Add1/2
  Switch1/1 -> Gain/1
  Constant2/1 -> Switch/3
  Constant3/1 -> Switch1/1
  Integrator/1 -> Saturation/1
  Gain1/1 -> Integrator/1
  Gain/1 -> Add1/1
  Constant1/1 -> Switch1/3

== system c00006M_harness/M096/Tank3/Control ==
  note: 1: Maintenance
      | 2: Reference
      | 3: Manual
  ControlType : Inport
  StartMaintenance : Inport  Port=2
  ManualReference : Inport  Port=3
  Fill : Inport  Port=4
  Empty : Inport  Port=5
  EmergencyButton : Inport  Port=6
  Temperature : Inport  Port=7
  LiquidLevel : Inport  Port=8
  Constant : Constant  Value=0
  Constant1 : Constant  Value=TempThreshold
  Logical Operator : Logic  Operator=OR  AllPortsSameDT=off  OutDataTypeStr=boolean
  Logical Operator1 : Logic  Operator=OR  AllPortsSameDT=off  OutDataTypeStr=boolean
  Maintenance : Subsystem
  ManualControlLiquidInOut : Subsystem
  ManualControlReference : Subsystem
  Multiport Switch : MultiPortSwitch
  Multiport Switch1 : MultiPortSwitch
  Relational Operator : RelationalOperator  Operator=>  OutDataTypeStr=boolean  RndMeth=Simplest
  Switch : Switch  Criteria=u2 > Threshold
  Switch1 : Switch  Criteria=u2 > Threshold
  LiquidIn : Outport
  LiquidOut : Outport  Port=2
  wires:
  Multiport Switch/1 -> Switch/3
  Multiport Switch1/1 -> Switch1/3
  ControlType/1 -> Multiport Switch1/1, Multiport Switch/1, Maintenance/1(Type)
  Maintenance/1(LiquidIn) -> Multiport Switch/2
  ManualControlReference/1(LiquidIn) -> Multiport Switch/3
  Maintenance/2(LiquidOut) -> Multiport Switch1/2
  ManualControlReference/2(LiquidOut) -> Multiport Switch1/3
  ManualReference/1 -> ManualControlReference/1(ManualReference)
  LiquidLevel/1 -> ManualControlLiquidInOut/3(LiquidLevel), ManualControlReference/2(LiquidLevel), Maintenance/3(LiquidLevel)
  ManualControlLiquidInOut/1(LiquidIn) -> Multiport Switch/4
  ManualControlLiquidInOut/2(LiquidOut) -> Multiport Switch1/4
  Empty/1 -> ManualControlLiquidInOut/2(Empty)
  Fill/1 -> ManualControlLiquidInOut/1(Fill)
  StartMaintenance/1 -> Maintenance/2(StartMaintenance)
  Switch/1 -> LiquidIn/1
  Switch1/1 -> LiquidOut/1
  Constant/1 -> Switch1/1, Switch/1
  EmergencyButton/1 -> Logical Operator/1, Logical Operator1/1
  Relational Operator/1 -> Logical Operator1/2, Logical Operator/2
  Logical Operator/1 -> Switch1/2
  Logical Operator1/1 -> Switch/2
  Temperature/1 -> Relational Operator/1
  Constant1/1 -> Relational Operator/2

== system c00006M_harness/M096/Tank3/MasterTankControl ==
  note: Priority tank must always have more liquid than others
  LiquidTank2 : Inport
  LiquidTank3 : Inport  Port=2
  Constant : Constant  Value=PriorityTank
  Constant1 : Constant  Value=false
  Logical Operator : Logic  Operator=NOT  AllPortsSameDT=off  OutDataTypeStr=boolean
  Multiport Switch : MultiPortSwitch
  Relational Operator1 : RelationalOperator  OutDataTypeStr=boolean  RndMeth=Simplest
  AllowTheTankFilling : Outport
  wires:
  Constant/1 -> Multiport Switch/1
  Relational Operator1/1 -> Multiport Switch/3
  Constant1/1 -> Multiport Switch/4, Multiport Switch/2
  Multiport Switch/1 -> Logical Operator/1
  Logical Operator/1 -> AllowTheTankFilling/1
  LiquidTank2/1 -> Relational Operator1/2
  LiquidTank3/1 -> Relational Operator1/1

== system c00006M_harness/M096/Tank3/TankModel ==
  LiquidIn : Inport
  LiquidOut : Inport  Port=2
  Add1 : Sum  Inputs=+-
  Constant1 : Constant  Value=0
  Constant2 : Constant  Value=0
  Constant3 : Constant
  Gain : Gain  Gain=1/R1
  Gain1 : Gain  Gain=1/A1
  Gain2 : Gain  Gain=1/R2
  Integrator : Integrator
  Saturation : Saturate  UpperLimit=hmax  LowerLimit=0
  Switch : Switch  Criteria=u2 ~= 0
  Switch1 : Switch  Criteria=u2 ~= 0
  LiquidLevel : Outport
  wires:
  Saturation/1 -> LiquidLevel/1, Gain2/1
  LiquidOut/1 -> Switch/2
  Add1/1 -> Gain1/1
  Gain2/1 -> Switch/1
  LiquidIn/1 -> Switch1/2
  Switch/1 -> Add1/2
  Switch1/1 -> Gain/1
  Constant2/1 -> Switch/3
  Constant3/1 -> Switch1/1
  Integrator/1 -> Saturation/1
  Gain1/1 -> Integrator/1
  Gain/1 -> Add1/1
  Constant1/1 -> Switch1/3

== system c00006M_harness/M097/Tank2/Control ==
  note: 1: Maintenance
      | 2: Reference
      | 3: Manual
  ControlType : Inport
  StartMaintenance : Inport  Port=2
  ManualReference : Inport  Port=3
  Fill : Inport  Port=4
  Empty : Inport  Port=5
  EmergencyButton : Inport  Port=6
  Temperature : Inport  Port=7
  LiquidLevel : Inport  Port=8
  Constant : Constant  Value=0
  Constant1 : Constant  Value=TempThreshold
  Logical Operator : Logic  Operator=OR  AllPortsSameDT=off  OutDataTypeStr=boolean
  Logical Operator1 : Logic  Operator=OR  AllPortsSameDT=off  OutDataTypeStr=boolean
  Maintenance : Subsystem
  ManualControlLiquidInOut : Subsystem
  ManualControlReference : Subsystem
  Multiport Switch : MultiPortSwitch
  Multiport Switch1 : MultiPortSwitch
  Relational Operator : RelationalOperator  Operator=>  OutDataTypeStr=boolean  RndMeth=Simplest
  Switch : Switch  Criteria=u2 > Threshold
  Switch1 : Switch  Criteria=u2 > Threshold
  LiquidIn : Outport
  LiquidOut : Outport  Port=2
  wires:
  Multiport Switch/1 -> Switch/3
  Multiport Switch1/1 -> Switch1/3
  ControlType/1 -> Multiport Switch1/1, Multiport Switch/1, Maintenance/1(Type)
  Maintenance/1(LiquidIn) -> Multiport Switch/2
  ManualControlReference/1(LiquidIn) -> Multiport Switch/3
  Maintenance/2(LiquidOut) -> Multiport Switch1/2
  ManualControlReference/2(LiquidOut) -> Multiport Switch1/3
  ManualReference/1 -> ManualControlReference/1(ManualReference)
  LiquidLevel/1 -> ManualControlLiquidInOut/3(LiquidLevel), ManualControlReference/2(LiquidLevel), Maintenance/3(LiquidLevel)
  ManualControlLiquidInOut/1(LiquidIn) -> Multiport Switch/4
  ManualControlLiquidInOut/2(LiquidOut) -> Multiport Switch1/4
  Empty/1 -> ManualControlLiquidInOut/2(Empty)
  Fill/1 -> ManualControlLiquidInOut/1(Fill)
  StartMaintenance/1 -> Maintenance/2(StartMaintenance)
  Switch/1 -> LiquidIn/1
  Switch1/1 -> LiquidOut/1
  Constant/1 -> Switch1/1, Switch/1
  EmergencyButton/1 -> Logical Operator/1, Logical Operator1/1
  Relational Operator/1 -> Logical Operator1/2, Logical Operator/2
  Logical Operator/1 -> Switch1/2
  Logical Operator1/1 -> Switch/2
  Temperature/1 -> Relational Operator/1
  Constant1/1 -> Relational Operator/2

== system c00006M_harness/M097/Tank2/MasterTankControl ==
  note: Priority tank must always have more liquid than others
  LiquidTank2 : Inport
  LiquidTank3 : Inport  Port=2
  Constant : Constant  Value=PriorityTank
  Constant1 : Constant  Value=false
  Logical Operator : Logic  Operator=NOT  AllPortsSameDT=off  OutDataTypeStr=boolean
  Multiport Switch : MultiPortSwitch
  Relational Operator1 : RelationalOperator  OutDataTypeStr=boolean  RndMeth=Simplest
  AllowTheTankFilling : Outport
  wires:
  LiquidTank2/1 -> Relational Operator1/1
  LiquidTank3/1 -> Relational Operator1/2
  Constant/1 -> Multiport Switch/1
  Relational Operator1/1 -> Multiport Switch/4
  Constant1/1 -> Multiport Switch/3, Multiport Switch/2
  Multiport Switch/1 -> Logical Operator/1
  Logical Operator/1 -> AllowTheTankFilling/1

== system c00006M_harness/M097/Tank2/TankModel ==
  LiquidIn : Inport
  LiquidOut : Inport  Port=2
  Add1 : Sum  Inputs=+-
  Constant1 : Constant  Value=0
  Constant2 : Constant  Value=0
  Constant3 : Constant
  Gain : Gain  Gain=1/R1
  Gain1 : Gain  Gain=1/A1
  Gain2 : Gain  Gain=1/R2
  Integrator : Integrator
  Saturation : Saturate  UpperLimit=hmax  LowerLimit=0
  Switch : Switch  Criteria=u2 ~= 0
  Switch1 : Switch  Criteria=u2 ~= 0
  LiquidLevel : Outport
  wires:
  Saturation/1 -> LiquidLevel/1, Gain2/1
  LiquidOut/1 -> Switch/2
  Add1/1 -> Gain1/1
  Gain2/1 -> Switch/1
  LiquidIn/1 -> Switch1/2
  Switch/1 -> Add1/2
  Switch1/1 -> Gain/1
  Constant2/1 -> Switch/3
  Constant3/1 -> Switch1/1
  Integrator/1 -> Saturation/1
  Gain1/1 -> Integrator/1
  Gain/1 -> Add1/1
  Constant1/1 -> Switch1/3

== system c00006M_harness/M097/Tank3/Control ==
  note: 1: Maintenance
      | 2: Reference
      | 3: Manual
  ControlType : Inport
  StartMaintenance : Inport  Port=2
  ManualReference : Inport  Port=3
  Fill : Inport  Port=4
  Empty : Inport  Port=5
  EmergencyButton : Inport  Port=6
  Temperature : Inport  Port=7
  LiquidLevel : Inport  Port=8
  Constant : Constant  Value=0
  Constant1 : Constant  Value=TempThreshold
  Logical Operator : Logic  Operator=OR  AllPortsSameDT=off  OutDataTypeStr=boolean
  Logical Operator1 : Logic  Operator=OR  AllPortsSameDT=off  OutDataTypeStr=boolean
  Maintenance : Subsystem
  ManualControlLiquidInOut : Subsystem
  ManualControlReference : Subsystem
  Multiport Switch : MultiPortSwitch
  Multiport Switch1 : MultiPortSwitch
  Relational Operator : RelationalOperator  Operator=>  OutDataTypeStr=boolean  RndMeth=Simplest
  Switch : Switch  Criteria=u2 > Threshold
  Switch1 : Switch  Criteria=u2 > Threshold
  LiquidIn : Outport
  LiquidOut : Outport  Port=2
  wires:
  Multiport Switch/1 -> Switch/3
  Multiport Switch1/1 -> Switch1/3
  ControlType/1 -> Multiport Switch1/1, Multiport Switch/1, Maintenance/1(Type)
  Maintenance/1(LiquidIn) -> Multiport Switch/2
  ManualControlReference/1(LiquidIn) -> Multiport Switch/3
  Maintenance/2(LiquidOut) -> Multiport Switch1/2
  ManualControlReference/2(LiquidOut) -> Multiport Switch1/3
  ManualReference/1 -> ManualControlReference/1(ManualReference)
  LiquidLevel/1 -> ManualControlLiquidInOut/3(LiquidLevel), ManualControlReference/2(LiquidLevel), Maintenance/3(LiquidLevel)
  ManualControlLiquidInOut/1(LiquidIn) -> Multiport Switch/4
  ManualControlLiquidInOut/2(LiquidOut) -> Multiport Switch1/4
  Empty/1 -> ManualControlLiquidInOut/2(Empty)
  Fill/1 -> ManualControlLiquidInOut/1(Fill)
  StartMaintenance/1 -> Maintenance/2(StartMaintenance)
  Switch/1 -> LiquidIn/1
  Switch1/1 -> LiquidOut/1
  Constant/1 -> Switch1/1, Switch/1
  EmergencyButton/1 -> Logical Operator/1, Logical Operator1/1
  Relational Operator/1 -> Logical Operator1/2, Logical Operator/2
  Logical Operator/1 -> Switch1/2
  Logical Operator1/1 -> Switch/2
  Temperature/1 -> Relational Operator/1
  Constant1/1 -> Relational Operator/2

== system c00006M_harness/M097/Tank3/MasterTankControl ==
  note: Priority tank must always have more liquid than others
  LiquidTank2 : Inport
  LiquidTank3 : Inport  Port=2
  Constant : Constant  Value=PriorityTank
  Constant1 : Constant  Value=false
  Logical Operator : Logic  Operator=NOT  AllPortsSameDT=off  OutDataTypeStr=boolean
  Multiport Switch : MultiPortSwitch
  Relational Operator1 : RelationalOperator  OutDataTypeStr=boolean  RndMeth=Simplest
  AllowTheTankFilling : Outport
  wires:
  Constant/1 -> Multiport Switch/1
  Relational Operator1/1 -> Multiport Switch/3
  Constant1/1 -> Multiport Switch/4, Multiport Switch/2
  Multiport Switch/1 -> Logical Operator/1
  Logical Operator/1 -> AllowTheTankFilling/1
  LiquidTank2/1 -> Relational Operator1/2
  LiquidTank3/1 -> Relational Operator1/1

== system c00006M_harness/M097/Tank3/TankModel ==
  LiquidIn : Inport
  LiquidOut : Inport  Port=2
  Add1 : Sum  Inputs=+-
  Constant1 : Constant  Value=0
  Constant2 : Constant  Value=0
  Constant3 : Constant
  Gain : Gain  Gain=1/R1
  Gain1 : Gain  Gain=1/A1
  Gain2 : Gain  Gain=1/R2
  Integrator : Integrator
  Saturation : Saturate  UpperLimit=hmax  LowerLimit=0
  Switch : Switch  Criteria=u2 ~= 0
  Switch1 : Switch  Criteria=u2 ~= 0
  LiquidLevel : Outport
  wires:
  Saturation/1 -> LiquidLevel/1, Gain2/1
  LiquidOut/1 -> Switch/2
  Add1/1 -> Gain1/1
  Gain2/1 -> Switch/1
  LiquidIn/1 -> Switch1/2
  Switch/1 -> Add1/2
  Switch1/1 -> Gain/1
  Constant2/1 -> Switch/3
  Constant3/1 -> Switch1/1
  Integrator/1 -> Saturation/1
  Gain1/1 -> Integrator/1
  Gain/1 -> Add1/1
  Constant1/1 -> Switch1/3
